simulink model "YAW_double_loop_ctrl"  (R2014a)
settings: Solver=ode45  StartTime=0.0  StopTime=1  RelTol=1e-3
libraries: simulink x2
settings Model: Creator=Felix  LastModifiedBy=Felix

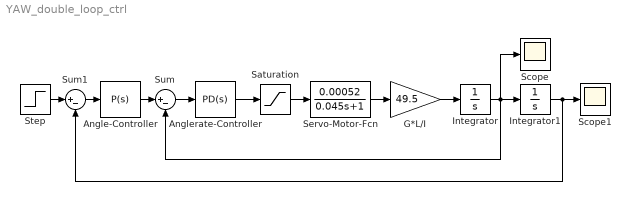
== system YAW_double_loop_ctrl ==
  Angle-Controller : simulink/Continuous/PID Controller  Controller=P  TimeDomain=Continuous-time  SampleTime=1  IntegratorMethod=Forward Euler  FilterMethod=Forward Euler  Form=Parallel  P=12  I=0  D=0  N=100  InitialConditionSource=internal  InitialConditionForIntegrator=0  InitialConditionForFilter=0  ExternalReset=none  LimitOutput=off  UpperSaturationLimit=inf  LowerSaturationLimit=-inf  LinearizeAsGain=on  AntiWindupMode=none  Kb=1  TrackingMode=off  Kt=1  PParamMin=[]  PParamMax=[]  PParamDataTypeStr=double  IParamMin=[]  IParamMax=[]  IParamDataTypeStr=double  DParamMin=[]  DParamMax=[]  NParamMin=[]  NParamMax=[]  KbParamMin=[]  KbParamMax=[]  KtParamMin=[]  KtParamMax=[]  POutMin=[]  POutMax=[]  POutDataTypeStr=double  IOutMin=[]  IOutMax=[]  IOutDataTypeStr=double  DOutMin=[]  DOutMax=[]  NOutMin=[]  NOutMax=[]  KbOutMin=[]  KbOutMax=[]  KtOutMin=[]  KtOutMax=[]  IntegratorOutMin=[]  IntegratorOutMax=[]  IntegratorOutDataTypeStr=single  FilterOutMin=[]  FilterOutMax=[]  SumOutMin=[]  SumOutMax=[]  SumOutDataTypeStr=double  SumI1OutMin=[]  SumI1OutMax=[]  SumI2OutMin=[]  SumI2OutMax=[]  SumI3OutMin=[]  SumI3OutMax=[]  SumDOutMin=[]  SumDOutMax=[]  SumAccumDataTypeStr=double  SaturationOutMin=[]  SaturationOutMax=[]  IntegratorContinuousStateAttributes=''  IntegratorStateMustResolveToSignalObject=off  IntegratorRTWStateStorageClass=Auto  FilterContinuousStateAttributes=''  FilterStateMustResolveToSignalObject=off  FilterRTWStateStorageClass=Auto
  Anglerate-Controller : simulink/Continuous/PID Controller  Controller=PD  TimeDomain=Continuous-time  SampleTime=1  IntegratorMethod=Forward Euler  FilterMethod=Forward Euler  Form=Parallel  P=2800  I=0  D=55  N=100  InitialConditionSource=internal  InitialConditionForIntegrator=0  InitialConditionForFilter=0  ExternalReset=none  LimitOutput=off  UpperSaturationLimit=inf  LowerSaturationLimit=-inf  LinearizeAsGain=on  AntiWindupMode=none  Kb=1  TrackingMode=off  Kt=1  PParamMin=[]  PParamMax=[]  PParamDataTypeStr=double  IParamMin=[]  IParamMax=[]  DParamMin=[]  DParamMax=[]  DParamDataTypeStr=double  NParamMin=[]  NParamMax=[]  NParamDataTypeStr=double  KbParamMin=[]  KbParamMax=[]  KtParamMin=[]  KtParamMax=[]  POutMin=[]  POutMax=[]  POutDataTypeStr=double  IOutMin=[]  IOutMax=[]  DOutMin=[]  DOutMax=[]  DOutDataTypeStr=double  NOutMin=[]  NOutMax=[]  NOutDataTypeStr=double  KbOutMin=[]  KbOutMax=[]  KtOutMin=[]  KtOutMax=[]  IntegratorOutMin=[]  IntegratorOutMax=[]  FilterOutMin=[]  FilterOutMax=[]  FilterOutDataTypeStr=single  SumOutMin=[]  SumOutMax=[]  SumOutDataTypeStr=double  SumI1OutMin=[]  SumI1OutMax=[]  SumI2OutMin=[]  SumI2OutMax=[]  SumI3OutMin=[]  SumI3OutMax=[]  SumDOutMin=[]  SumDOutMax=[]  SumDOutDataTypeStr=double  SumAccumDataTypeStr=double  SumDAccumDataTypeStr=double  SaturationOutMin=[]  SaturationOutMax=[]  IntegratorContinuousStateAttributes=''  IntegratorStateMustResolveToSignalObject=off  IntegratorRTWStateStorageClass=Auto  FilterContinuousStateAttributes=''  FilterStateMustResolveToSignalObject=off  FilterRTWStateStorageClass=Auto
  G*L/I : Gain  Gain=49.5
  Integrator : Integrator
  Integrator1 : Integrator
  Saturation : Saturate  UpperLimit=3000  LowerLimit=-3000
  Scope : Scope
  Scope1 : Scope
      settings: TimeRange=1.5  YMin=-1.045075125208682  YMax=-1.031719532554258
  Servo-Motor-Fcn : TransferFcn  Numerator=[0.00052]  Denominator=[0.045 1]
  Step : Step  Time=0.2  SampleTime=0
  Sum : Sum  Inputs=|+-
  Sum1 : Sum  Inputs=|+-
  wires:
  Sum1/1 -> Angle-Controller/1
  Servo-Motor-Fcn/1 -> G*L/I/1
  G*L/I/1 -> Integrator/1
  Integrator/1 -> Integrator1/1, Scope/1, Sum/2
  Integrator1/1 -> Sum1/2, Scope1/1
  Sum/1 -> Anglerate-Controller/1
  Anglerate-Controller/1 -> Saturation/1
  Saturation/1 -> Servo-Motor-Fcn/1
  Step/1 -> Sum1/1
  Angle-Controller/1 -> Sum/1
